simulink model "Model"  (R2024b)
settings: Solver=FixedStepAuto  StartTime=0.0  StopTime=17  FixedStep=0.001  RelTol=1e-3
values from neighbouring files (symbols this model uses):
  A_8 = 0.07    [Dane.m]
  C_Beta_vec = linspace(0, 1, beta_points)    [generate_maps.m]    (also in mapy_new.m = [0, 0.25, 0.5, 0.75, 1.0])
  C_Eff_map = zeros(n_points, beta_points)    [generate_maps.m]    (also in mapy_new.m = [)
  c_H = Ma*sqrt(R*kappa*T_H)    [Dane.m]
  C_Nc_vec = linspace(0.5, 1.05, n_points)    [generate_maps.m]    (also in mapy_new.m = [0.5, 0.8, 0.9, 1.0, 1.05])
  C_PR_map = zeros(n_points, beta_points)    [generate_maps.m]    (also in mapy_new.m = [)
  C_Wc_map = zeros(n_points, beta_points)    [generate_maps.m]    (also in mapy_new.m = [)
  cp = 1005    [Dane.m]
  cp_sp = 1152    [Dane.m]
  eta_c_nom = 0.78    [Dane.m]
  J = 5    [Dane.m]
  kappa = 1.4    [Dane.m]
  kappa_sp = 1.33    [Dane.m]
  m_dot_nom = 4.5    [Dane.m]
  Ma = 0.5    [Dane.m]
  n_nom = 41000    [Dane.m]
  p_0 = 101325    [Dane.m]
  p_H = p_0*(1-H/44300)^5.256    (= 53994.0459955)    [Dane.m]
  phi_d = 0.98    [Dane.m]
  pi_c_nom = 5.8    [Dane.m]
  pi_ks = 0.95    [Dane.m]
  R = 288    [Dane.m]
  sigma_rw = 1    [Dane.m]
  sigma_wl = 0.95    [Dane.m]
  T_0 = 288.15    [Dane.m]
  T_Eff_map = zeros(n_points, n_points)    [generate_maps.m]    (also in mapy_new.m = [)
  T_Nc_vec = linspace(0.5, 1.05, n_points)    [generate_maps.m]    (also in mapy_new.m = [0.5, 0.8, 0.9, 1.0, 1.05])
  T_PR_vec = linspace(1.2, 3.5, n_points)    [generate_maps.m]    (also in mapy_new.m = [1.5, 2.0, 2.5, 3.0, 3.5])
  T_Wc_map = zeros(n_points, n_points)    [generate_maps.m]    (also in mapy_new.m = [)
  W = 43*10^6    (= 43000000)    [Dane.m]
undefined symbols (not defined in the file or in its folder): m_dot
libraries: mpclib x1, slpidlib x1
settings Model: Creator=mordw  LastModifiedBy=mordw

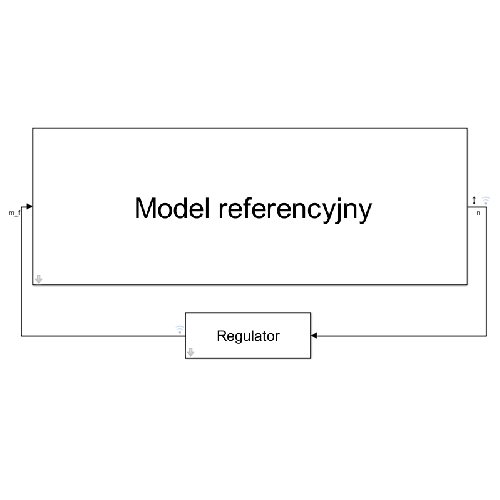
[thumbnail: Simulink's stored preview of the top-level diagram]
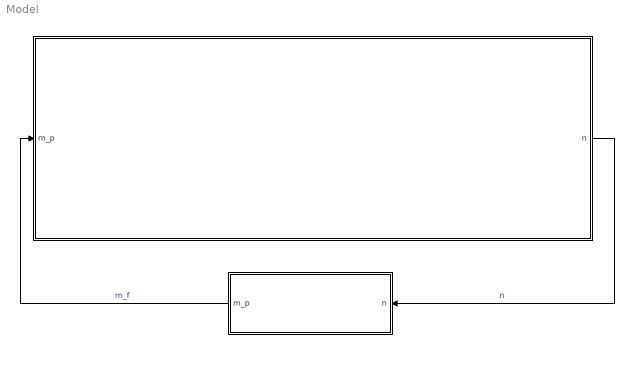
== system Model ==
  " " : Subsystem
      mask DialogControl Control2 Prompt: Reference model
  "  " : Subsystem
  wires:
  " "/1(n) -> "  "/1(n)  "n"
  "  "/1(m_p) -> " "/1(m_p)  "m_f"

== system Model/  ==
  m_p : Inport
  Reference dobry : Subsystem
  Terminator : Terminator  Commented=on
  Terminator1 : Terminator  Commented=on
  Terminator2 : Terminator  Commented=on
  n : Outport
  wires:
  m_p/1 -> Reference dobry/1(m_p1)
  Reference dobry/1(n1) -> n/1

== system Model/   ==
  n : Inport
  Constant : Constant  Commented=on  Value=n_nom
  Constant1 : Constant  Value=n_nom
  Constant2 : Constant
  MPC Controller : mpclib/MPC Controller  Commented=on  SCDEnableBlockLinearizationSpecification=on  mpcobj=mpc_controller  is_multiple=0  enable_value=0  return_u0=off  updateMPCinCallerWorkspace=on  md_inport=off  mv_inport=off  uref_inport=off  return_cost=off  return_mvseq=off  return_qpstatus=off  return_xseq=off  return_state=off  return_ovseq=off  state_inport=off  umin_inport=off  umax_inport=off  ymin_inport=off  ymax_inport=off  cc_inport=off  ywt_inport=off  uwt_inport=off  duwt_inport=off  rhoeps_inport=off  pm_inport=off  MaximumP=10  HorizonChoice=FixedHorizon  n_ts=0.01  n_p=50  n_mv=1  n_md=0  n_ud=0  n_mo=1  n_uo=0  BlockDataType=double  SampleTimeInherited=off  switch_inport=off
  PID Controller : slpidlib/PID Controller  Controller=PID  Form=Parallel  TimeDomain=Continuous-time  UseExternalTs=off  SampleTime=-1  IntegratorMethod=Forward Euler  FilterMethod=Forward Euler  ControllerParametersSource=internal  P=0.01  I=0.005  UseKiTs=off  D=0  UseExternalDerivativeSource=off  N=100  UseFilter=on  TunerSelectOption=Transfer Function Based (PID Tuner App)  InitialConditionSource=internal  InitialConditionForIntegrator=0  InitialConditionForFilter=0  DifferentiatorICPrevScaledInput=0  ExternalReset=none  TrackingMode=off  Kt=1  LimitOutput=on  SatLimitsSource=internal  UpperSaturationLimit=0.5  LowerSaturationLimit=0  LinearizeAsGain=on  AntiWindupMode=back-calculation  Kb=5  LimitIntegrator=off  UpperIntegratorSaturationLimit=inf  LowerIntegratorSaturationLimit=-inf  POutMin=[]  POutMax=[]  IOutMin=[]  IOutMax=[]  DOutMin=[]  DOutMax=[]  NOutMin=[]  NOutMax=[]  SumOutMin=[]  SumOutMax=[]  SaturationOutMin=[]  SaturationOutMax=[]  PParamMin=[]  PParamMax=[]  IParamMin=[]  IParamMax=[]  DParamMin=[]  DParamMax=[]  NParamMin=[]  NParamMax=[]  KbParamMin=[]  KbParamMax=[]  KtParamMin=[]  KtParamMax=[]  KbOutMin=[]  KbOutMax=[]  KtOutMin=[]  KtOutMax=[]  IntegratorOutMin=[]  IntegratorOutMax=[]  FilterOutMin=[]  FilterOutMax=[]  SumI1OutMin=[]  SumI1OutMax=[]  SumI2OutMin=[]  SumI2OutMax=[]  SumI3OutMin=[]  SumI3OutMax=[]  SumI4OutMin=[]  SumI4OutMax=[]  SumDOutMin=[]  SumDOutMax=[]  DifferentiatorOutMin=[]  DifferentiatorOutMax=[]  FilterDiffOutCoefMin=[]  FilterDiffOutCoefMax=[]  ReciprocalOutMin=[]  ReciprocalOutMax=[]  SumDenOutMin=[]  SumDenOutMax=[]  SumNumOutMin=[]  SumNumOutMax=[]  DivideOutMin=[]  DivideOutMax=[]  UdiffTsProdOutMin=[]  UdiffTsProdOutMax=[]  NTsProdOutMin=[]  NTsProdOutMax=[]  UintegralTsProdOutMin=[]  UintegralTsProdOutMax=[]  UngainTsProdOutMin=[]  UngainTsProdOutMax=[]  ClampingZeroOutDataTypeStr=Inherit: Inherit via back propagation  ClampingZeroOutMin=[]  ClampingZeroOutMax=[]  FilterDenConstantOutDataTypeStr=Inherit: Inherit via back propagation  FilterDenConstantOutMin=[]  FilterDenConstantOutMax=[]  PCopyOutDataTypeStr=Inherit: Inherit via back propagation  PCopyOutMin=[]  PCopyOutMax=[]  NCopyOutDataTypeStr=Inherit: Inherit via back propagation  NCopyOutMin=[]  NCopyOutMax=[]  IntegratorContinuousStateAttributes=''  IntegratorStateMustResolveToSignalObject=off  IntegratorRTWStateStorageClass=Auto  FilterContinuousStateAttributes=''  FilterStateMustResolveToSignalObject=off  FilterRTWStateStorageClass=Auto  ParallelPVariant=InternalParameters  IdealPVariant=Disabled  IVariant=InternalParameters  DVariant=InternalParameters  IntegratorVariant=Continuous  SatVariant=Enabled  AWVariant=BackCalculation  PCopyVariant=Disabled  TRVariant=Disabled  FdbkBlocksVariant=Forward  IdealPFdbkVariant=Disabled  SatFdbkVariant=Disabled  DerivativeFilterVariant=ContFilter  NVariant=InternalParameters  NCopyVariant=Disabled  FilterICVariant=InternalICsFilter  IntegratorICVariant=InternalICs  ExternalResetVariant=Disabled  TRSumVariant=Passthrough  SumFdbkVariant=Disabled  SumVariant=Sum_PID  TsampFilterVariant=InternalTs  TsampNgainVariant=Passthrough  TsampIntegralVariant=Disabled_SignalSpec  ExternalSaturationOutDataTypeStr=Inherit: Same as second input  DerivativeSourceVariant=ErrorSignal  PreIntVariant=InternalPreInt
  Sum : Sum  Inputs=|-+
  Switch : Switch  Criteria=u2 > Threshold  SaturateOnIntegerOverflow=off  InputSameDT=off
  m_p : Outport
  wires:
  n/1 -> Sum/1, MPC Controller/1
  PID Controller/1 -> Switch/1
  MPC Controller/1 -> Switch/3
  Constant1/1 -> Sum/2
  Constant/1 -> MPC Controller/2
  Sum/1 -> PID Controller/1
  Constant2/1 -> Switch/2
  Switch/1 -> m_p/1  "m_p"

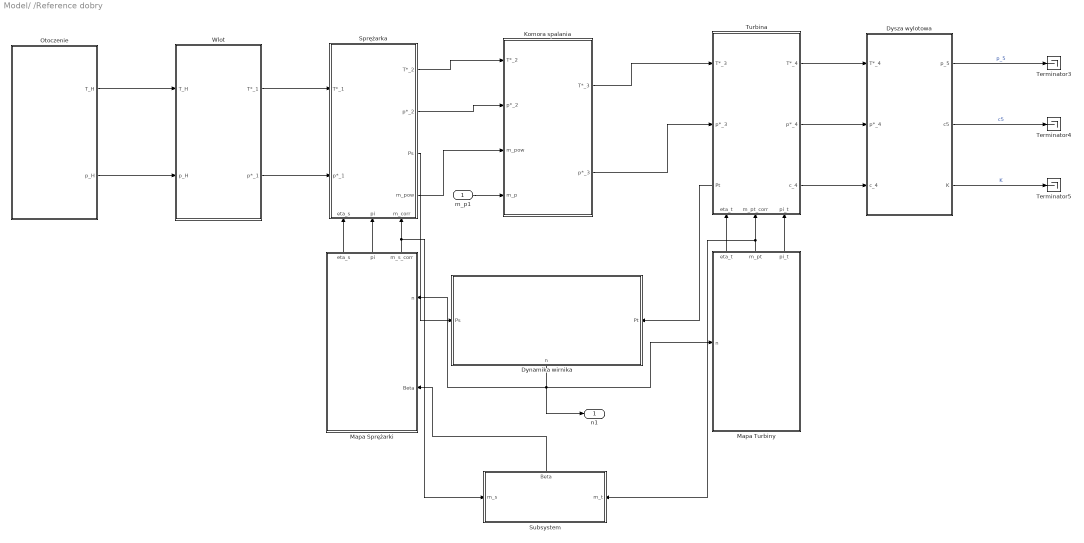
== system Model/ /Reference dobry ==
  m_p1 : Inport
  Dynamika wirnika : Subsystem
      settings: PortSchema="{\"entries\":[{\"content\":{\"sides\":[{\"content\":{\"connectorIds\":[\"In1\"]},\"type\":\"ConnectorPlacement.EquallySpacedRectSide\",\"uuid\":\"92648d91-603a-470e-8d2a-f02149c3db38\"},{\"content\":{\"connectorIds\":[\"In2\"],\"side\":\"RIGHT\"},\"type\":\"ConnectorPlacement.EquallySpacedRectSide\",\"uuid\":\"414f3566-06b2-4981-8d9f-99d3b0ae2fa9\"},{\"content\":{\"side\":\"TOP\"},\"type\":\"ConnectorPlacement.EquallySpacedRectSide\",\"uuid\":\"127541e1-5e00-46d2-b9c4-1484edc24234\"},{\"content\":{\"connectorIds\":[\"Out1\"],\"side\":\"BOTTOM\"},\"type\":\"ConnectorPlacement.EquallySpacedRectSide\",\"uuid\":\"a5106de6-ce0f-46b5-8051-6428c4816053\"}]},\"type\":\"ConnectorPlacement.EquallySpacedConnector\",\"uuid\":\"41cf9bbd-cf38-41c3-a622-f9a01faf9b59\"}],\"packageUris\":[\"http://schema.mathworks.com/mf0/Connector/R2020b\"],\"version\":\"1.0\"}"
  Dysza wylotowa : Subsystem
  Komora spalania : Subsystem
  Mapa Sprężarki : Subsystem
      settings: PortSchema="{\"entries\":[{\"content\":{\"sides\":[{\"content\":{},\"type\":\"ConnectorPlacement.EquallySpacedRectSide\",\"uuid\":\"8677f900-7922-4478-aeeb-e88a17ef6356\"},{\"content\":{\"connectorIds\":[\"In1\",\"In2\"],\"side\":\"RIGHT\"},\"type\":\"ConnectorPlacement.EquallySpacedRectSide\",\"uuid\":\"8ac603c2-697e-40fb-a61e-8eac1944f047\"},{\"content\":{\"connectorIds\":[\"Out1\",\"Out2\",\"Out3\"],\"side\":\"TOP\"},\"type\":\"ConnectorPlacement.EquallySpacedRectSide\",\"uuid\":\"1291509f-f986-4666-8166-1e03e99acc3f\"},{\"content\":{\"side\":\"BOTTOM\"},\"type\":\"ConnectorPlacement.EquallySpacedRectSide\",\"uuid\":\"87618aba-7d63-48a9-a830-8ed0b0805b31\"}]},\"type\":\"ConnectorPlacement.EquallySpacedConnector\",\"uuid\":\"5f7b5324-b2c0-4c4f-ba23-276b96a3be49\"}],\"packageUris\":[\"http://schema.mathworks.com/mf0/Connector/R2020b\"],\"version\":\"1.0\"}"
  Mapa Turbiny : Subsystem
      settings: PortSchema="{\"entries\":[{\"content\":{\"sides\":[{\"content\":{\"connectorIds\":[\"In1\"]},\"type\":\"ConnectorPlacement.EquallySpacedRectSide\",\"uuid\":\"5cf3ab21-3172-420e-8db2-451205a4f6d8\"},{\"content\":{\"side\":\"RIGHT\"},\"type\":\"ConnectorPlacement.EquallySpacedRectSide\",\"uuid\":\"e1f4544a-94e2-479d-8805-7e94a98bc078\"},{\"content\":{\"connectorIds\":[\"Out1\",\"Out2\",\"Out3\"],\"side\":\"TOP\"},\"type\":\"ConnectorPlacement.EquallySpacedRectSide\",\"uuid\":\"0d6b6710-b665-43c6-ac6f-8bcced33118f\"}]},\"type\":\"ConnectorPlacement.EquallySpacedConnector\",\"uuid\":\"393c9c26-fe71-43c8-a3ab-bf8cb9c23c8b\"}],\"packageUris\":[\"http://schema.mathworks.com/mf0/Connector/R2020b\"],\"version\":\"1.0\"}"
  Otoczenie : Subsystem
  Sprężarka : Subsystem
      settings: PortSchema="{\"entries\":[{\"content\":{\"sides\":[{\"content\":{\"connectorIds\":[\"In1\",\"In2\"]},\"type\":\"ConnectorPlacement.EquallySpacedRectSide\",\"uuid\":\"5ad9138f-573e-4bb6-8f90-45256150ad02\"},{\"content\":{\"connectorIds\":[\"Out1\",\"Out2\",\"Out3\",\"Out4\"],\"side\":\"RIGHT\"},\"type\":\"ConnectorPlacement.EquallySpacedRectSide\",\"uuid\":\"748e4777-2a7e-4826-9de5-35a340d0e0d9\"},{\"content\":{\"side\":\"TOP\"},\"type\":\"ConnectorPlacement.EquallySpacedRectSide\",\"uuid\":\"d6ba970d-5e85-4191-9407-cf63c790295c\"},{\"content\":{\"connectorIds\":[\"In3\",\"In4\",\"In5\"],\"side\":\"BOTTOM\"},\"type\":\"ConnectorPlacement.EquallySpacedRectSide\",\"uuid\":\"1930f8a7-28af-49c4-96e2-50b54aac2f51\"}]},\"type\":\"ConnectorPlacement.EquallySpacedConnector\",\"uuid\":\"98d1a612-9d3a-4741-82d1-8163c8f597bd\"}],\"packageUris\":[\"http://schema.mathworks.com/mf0/Connector/R2020b\"],\"version\":\"1.0\"}"
  Subsystem : Subsystem
      settings: PortSchema="{\"entries\":[{\"content\":{\"sides\":[{\"content\":{\"connectorIds\":[\"In1\"]},\"type\":\"ConnectorPlacement.EquallySpacedRectSide\",\"uuid\":\"a539ccee-3b56-4fd0-8aa8-8b3e66e9dd4a\"},{\"content\":{\"connectorIds\":[\"In2\"],\"side\":\"RIGHT\"},\"type\":\"ConnectorPlacement.EquallySpacedRectSide\",\"uuid\":\"8c1e68bc-092f-4324-808d-b2eeaf4424db\"},{\"content\":{\"connectorIds\":[\"Out1\"],\"side\":\"TOP\"},\"type\":\"ConnectorPlacement.EquallySpacedRectSide\",\"uuid\":\"5ad00f7f-de76-476d-96e9-8c0e667f1b36\"}]},\"type\":\"ConnectorPlacement.EquallySpacedConnector\",\"uuid\":\"625eb8fa-74b9-4e26-bcda-3b6095be352e\"}],\"packageUris\":[\"http://schema.mathworks.com/mf0/Connector/R2020b\"],\"version\":\"1.0\"}"
  Terminator3 : Terminator
  Terminator4 : Terminator
  Terminator5 : Terminator
  Turbina : Subsystem
      settings: PortSchema="{\"entries\":[{\"content\":{\"sides\":[{\"content\":{\"connectorIds\":[\"In1\",\"In2\",\"Out4\"]},\"type\":\"ConnectorPlacement.EquallySpacedRectSide\",\"uuid\":\"f4a9e5e5-b95d-47b8-93e5-cedd35d908d0\"},{\"content\":{\"connectorIds\":[\"Out1\",\"Out2\",\"Out3\"],\"side\":\"RIGHT\"},\"type\":\"ConnectorPlacement.EquallySpacedRectSide\",\"uuid\":\"10b6ea61-f01f-4e48-ad07-dc4cbfd91ff5\"},{\"content\":{\"side\":\"TOP\"},\"type\":\"ConnectorPlacement.EquallySpacedRectSide\",\"uuid\":\"208658a8-c4a1-42db-ac9c-b16758812c43\"},{\"content\":{\"connectorIds\":[\"In3\",\"In4\",\"In5\"],\"side\":\"BOTTOM\"},\"type\":\"ConnectorPlacement.EquallySpacedRectSide\",\"uuid\":\"fa42c5c3-0699-4620-9578-eed2ede52a20\"}]},\"type\":\"ConnectorPlacement.EquallySpacedConnector\",\"uuid\":\"0f96be96-72d8-41e4-aada-f9d1a25f1c70\"}],\"packageUris\":[\"http://schema.mathworks.com/mf0/Connector/R2020b\"],\"version\":\"1.0\"}"
  Wlot : Subsystem
  n1 : Outport
  wires:
  Komora spalania/2(p*_3) -> Turbina/2(p*_3)
  Komora spalania/1(T*_3) -> Turbina/1(T*_3)
  Mapa Turbiny/2(m_pt) -> Subsystem/2(m_t), Turbina/4(m_pt_corr)
  Otoczenie/2(p_H) -> Wlot/2(p_H)
  Dynamika wirnika/1(n) -> n1/1, Mapa Sprężarki/1(n), Mapa Turbiny/1(n)
  Turbina/4(Pt) -> Dynamika wirnika/2(Pt)
  Dysza wylotowa/2(c5) -> Terminator4/1  "c5"
  Mapa Turbiny/3(pi_t) -> Turbina/5(pi_t)
  Sprężarka/1(T*_2) -> Komora spalania/1(T*_2)
  Dysza wylotowa/1(p_5) -> Terminator3/1  "p_5"
  Mapa Sprężarki/2(pi) -> Sprężarka/4(pi)
  Dysza wylotowa/3(K) -> Terminator5/1  "K"
  Mapa Sprężarki/1(eta_s) -> Sprężarka/3(eta_s)
  Sprężarka/3(Ps) -> Dynamika wirnika/1(Ps)
  Turbina/3(c_4) -> Dysza wylotowa/3(c_4)
  Wlot/1(T*_1) -> Sprężarka/1(T*_1)
  Mapa Turbiny/1(eta_t) -> Turbina/3(eta_t)
  Turbina/1(T*_4) -> Dysza wylotowa/1(T*_4)
  Otoczenie/1(T_H) -> Wlot/1(T_H)
  Turbina/2(p*_4) -> Dysza wylotowa/2(p*_4)
  m_p1/1 -> Komora spalania/4(m_p)
  Wlot/2(p*_1) -> Sprężarka/2(p*_1)
  Sprężarka/2(p*_2) -> Komora spalania/2(p*_2)
  Mapa Sprężarki/3(m_s_corr) -> Subsystem/1(m_s), Sprężarka/5(m_corr)
  Sprężarka/4(m_pow) -> Komora spalania/3(m_pow)
  Subsystem/1(Beta) -> Mapa Sprężarki/2(Beta)

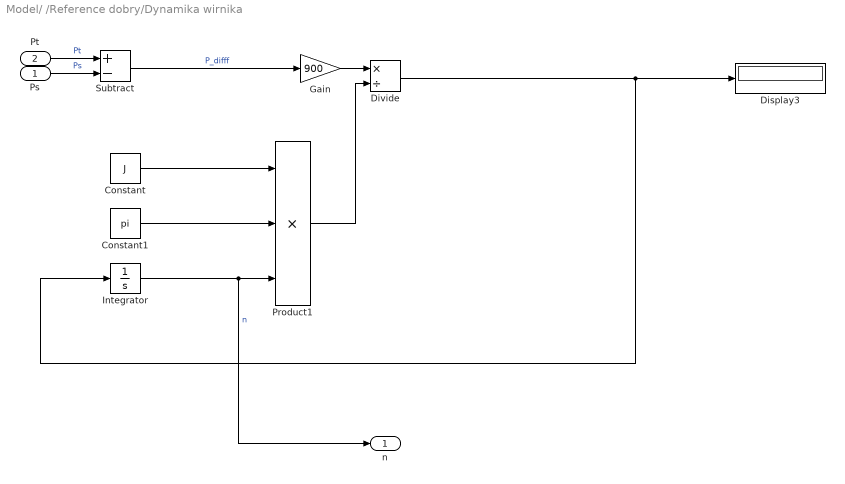
== system Model/ /Reference dobry/Dynamika wirnika ==
  Ps : Inport
  Pt : Inport  Port=2
  Constant : Constant  Value=J
  Constant1 : Constant  Value=pi
  Display3 : Display
  Divide : Product  Inputs=*/
  Gain : Gain  Gain=900
  Integrator : Integrator  InitialCondition=n_nom
  Product1 : Product  Inputs=3
  Subtract : Sum  Inputs=+-
  n : Outport
  wires:
  Integrator/1 -> n/1, Product1/3  "n"
  Divide/1 -> Integrator/1, Display3/1
  Pt/1 -> Subtract/1  "Pt"
  Subtract/1 -> Gain/1  "P_difff"
  Product1/1 -> Divide/2
  Constant1/1 -> Product1/2
  Constant/1 -> Product1/1
  Gain/1 -> Divide/1
  Ps/1 -> Subtract/2  "Ps"

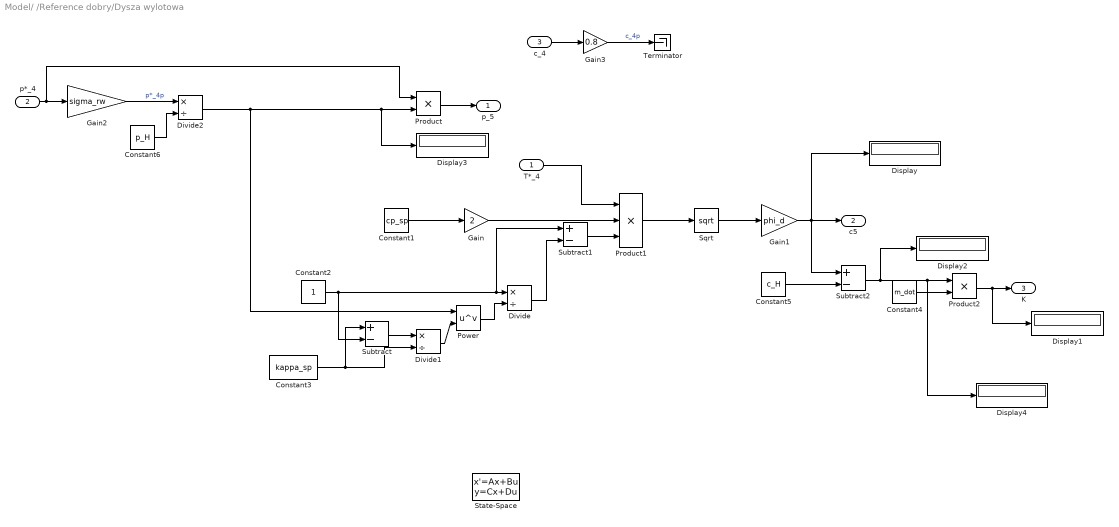
== system Model/ /Reference dobry/Dysza wylotowa ==
  T*_4 : Inport
  p*_4 : Inport  Port=2
  c_4 : Inport  Port=3
  Constant1 : Constant  Value=cp_sp
  Constant2 : Constant
  Constant3 : Constant  Value=kappa_sp
  Constant4 : Constant  Value=m_dot
  Constant5 : Constant  Value=c_H
  Constant6 : Constant  Value=p_H
  Display{,1..4} (5 alike) : Display
  Divide : Product  Inputs=*/
  Divide1 : Product  Inputs=*/
  Divide2 : Product  Inputs=*/
  Gain : Gain  Gain=2
  Gain1 : Gain  Gain=phi_d
  Gain2 : Gain  Gain=sigma_rw
  Gain3 : Gain  Gain=0.8
  Power : Math  Operator=pow
  Product : Product
  Product1 : Product  Inputs=3
  Product2 : Product
  Sqrt : Sqrt
  State-Space : StateSpace  InitialCondition=0
  Subtract : Sum  Inputs=+-
  Subtract1 : Sum  Inputs=+-
  Subtract2 : Sum  Inputs=+-
  Terminator : Terminator
  p_5 : Outport
  c5 : Outport  Port=2
  K : Outport  Port=3
  wires:
  Constant6/1 -> Divide2/2
  Gain3/1 -> Terminator/1  "c_4p"
  c_4/1 -> Gain3/1
  Gain2/1 -> Divide2/1  "p*_4p"
  Product2/1 -> K/1, Display1/1
  Subtract2/1 -> Product2/1, Display4/1, Display2/1
  Constant5/1 -> Subtract2/2
  Constant4/1 -> Product2/2
  Gain1/1 -> c5/1, Subtract2/1, Display/1
  Sqrt/1 -> Gain1/1
  Subtract1/1 -> Product1/3
  Divide/1 -> Subtract1/2
  Power/1 -> Divide/2
  Divide1/1 -> Power/2
  Subtract/1 -> Divide1/1
  Constant3/1 -> Subtract/1, Divide1/2
  Constant2/1 -> Subtract/2, Divide/1, Subtract1/1
  Product1/1 -> Sqrt/1
  T*_4/1 -> Product1/1
  Gain/1 -> Product1/2
  Constant1/1 -> Gain/1
  p*_4/1 -> Gain2/1, Product/1
  Divide2/1 -> Power/1, Product/2, Display3/1
  Product/1 -> p_5/1

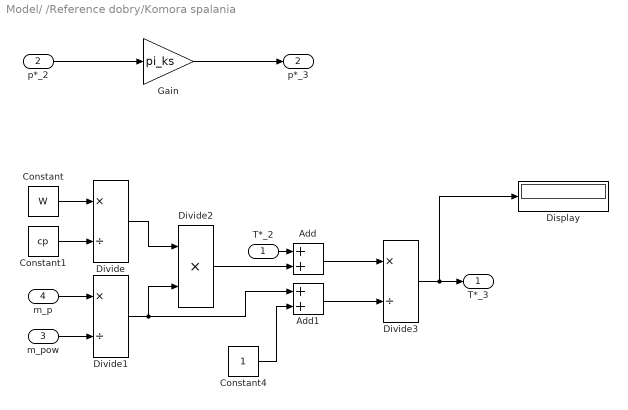
== system Model/ /Reference dobry/Komora spalania ==
  T*_2 : Inport
  p*_2 : Inport  Port=2
  m_pow : Inport  Port=3
  m_p : Inport  Port=4
  Add : Sum
  Add1 : Sum
  Constant : Constant  Value=W
  Constant1 : Constant  Value=cp
  Constant4 : Constant
  Display : Display
  Divide : Product  Inputs=*/
  Divide1 : Product  Inputs=*/
  Divide2 : Product  Inputs=**
  Divide3 : Product  Inputs=*/
  Gain : Gain  Gain=pi_ks
  T*_3 : Outport
  p*_3 : Outport  Port=2
  wires:
  m_p/1 -> Divide1/1
  Gain/1 -> p*_3/1
  p*_2/1 -> Gain/1
  Divide3/1 -> T*_3/1, Display/1
  Divide/1 -> Divide2/1
  Divide1/1 -> Divide2/2, Add1/1
  Constant4/1 -> Add1/2
  Add1/1 -> Divide3/2
  Add/1 -> Divide3/1
  T*_2/1 -> Add/1
  Divide2/1 -> Add/2
  m_pow/1 -> Divide1/2
  Constant1/1 -> Divide/2
  Constant/1 -> Divide/1

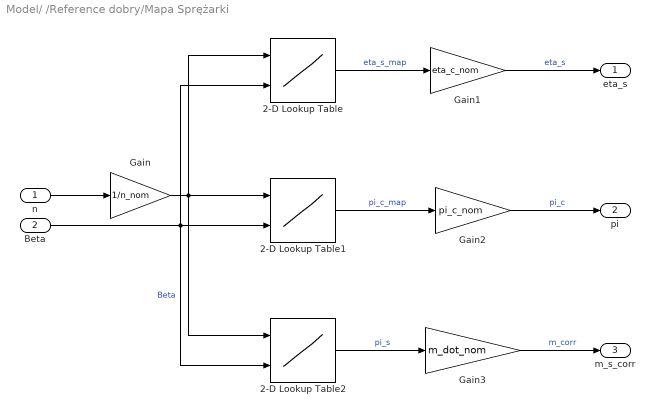
== system Model/ /Reference dobry/Mapa Sprężarki ==
  n : Inport
  Beta : Inport  Port=2
  2-D Lookup Table : Lookup_n-D  BreakpointsForDimension1=C_Nc_vec  BreakpointsForDimension2=C_Beta_vec  Table=C_Eff_map  InternalRulePriority=Speed  RndMeth=Simplest
      settings: InputPortMap=u0,u1
  2-D Lookup Table1 : Lookup_n-D  BreakpointsForDimension1=C_Nc_vec  BreakpointsForDimension2=C_Beta_vec  Table=C_PR_map  InternalRulePriority=Speed  RndMeth=Simplest
      settings: InputPortMap=u0,u1
  2-D Lookup Table2 : Lookup_n-D  BreakpointsForDimension1=C_Nc_vec  BreakpointsForDimension2=C_Beta_vec  Table=C_Wc_map  InternalRulePriority=Speed  RndMeth=Simplest
      settings: InputPortMap=u0,u1
  Gain : Gain  Gain=1/n_nom
  Gain1 : Gain  Gain=eta_c_nom
  Gain2 : Gain  Gain=pi_c_nom
  Gain3 : Gain  Gain=m_dot_nom
  eta_s : Outport
  pi : Outport  Port=2
  m_s_corr : Outport  Port=3
  wires:
  Gain/1 -> 2-D Lookup Table2/1, 2-D Lookup Table/1, 2-D Lookup Table1/1
  Beta/1 -> 2-D Lookup Table2/2, 2-D Lookup Table1/2, 2-D Lookup Table/2  "Beta"
  n/1 -> Gain/1
  2-D Lookup Table/1 -> Gain1/1  "eta_s_map"
  2-D Lookup Table1/1 -> Gain2/1  "pi_c_map"
  Gain1/1 -> eta_s/1  "eta_s"
  Gain2/1 -> pi/1  "pi_c"
  2-D Lookup Table2/1 -> Gain3/1  "pi_s"
  Gain3/1 -> m_s_corr/1  "m_corr"

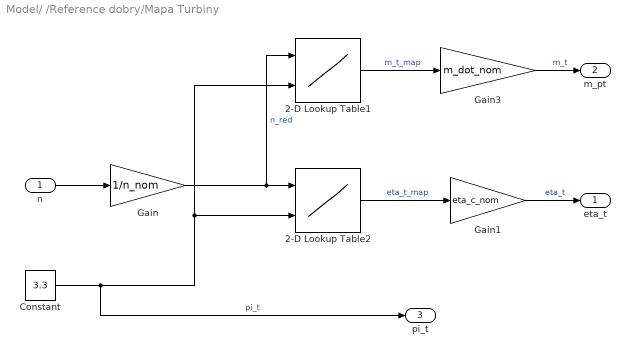
== system Model/ /Reference dobry/Mapa Turbiny ==
  n : Inport
  2-D Lookup Table1 : Lookup_n-D  BreakpointsForDimension1=T_Nc_vec  BreakpointsForDimension2=T_PR_vec  Table=T_Wc_map  InternalRulePriority=Speed  RndMeth=Simplest
      settings: InputPortMap=u0,u1
  2-D Lookup Table2 : Lookup_n-D  BreakpointsForDimension1=T_Nc_vec  BreakpointsForDimension2=T_PR_vec  Table=T_Eff_map  InternalRulePriority=Speed  RndMeth=Simplest
      settings: InputPortMap=u0,u1
  Constant : Constant  Value=3.3
  Gain : Gain  Gain=1/n_nom
  Gain1 : Gain  Gain=eta_c_nom
  Gain3 : Gain  Gain=m_dot_nom
  eta_t : Outport
  m_pt : Outport  Port=2
  pi_t : Outport  Port=3
  wires:
  2-D Lookup Table1/1 -> Gain3/1  "m_t_map"
  Gain/1 -> 2-D Lookup Table2/1, 2-D Lookup Table1/1  "n_red"
  2-D Lookup Table2/1 -> Gain1/1  "eta_t_map"
  n/1 -> Gain/1
  Constant/1 -> 2-D Lookup Table2/2, 2-D Lookup Table1/2, pi_t/1  "pi_t"
  Gain3/1 -> m_pt/1  "m_t"
  Gain1/1 -> eta_t/1  "eta_t"

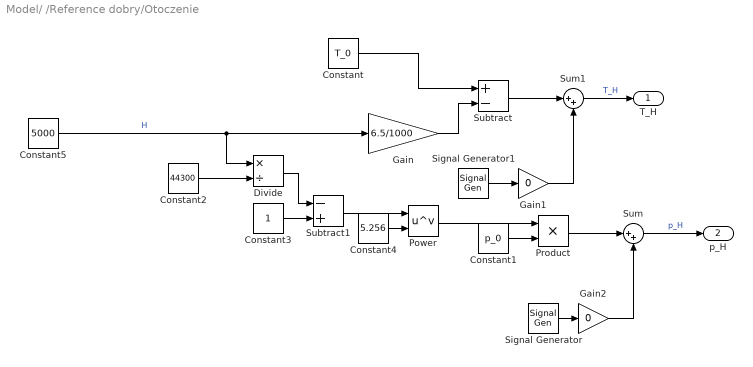
== system Model/ /Reference dobry/Otoczenie ==
  Constant : Constant  Value=T_0
  Constant1 : Constant  Value=p_0
  Constant2 : Constant  Value=44300
  Constant3 : Constant
  Constant4 : Constant  Value=5.256
  Constant5 : Constant  Value=5000
  Divide : Product  Inputs=*/
  Gain : Gain  Gain=6.5/1000
  Gain1 : Gain  Gain=0
  Gain2 : Gain  Gain=0
  Power : Math  Operator=pow
  Product : Product
  Signal Generator : SignalGenerator  WaveForm=square  Amplitude=5000  Frequency=0.5
  Signal Generator1 : SignalGenerator  Amplitude=15  Frequency=0.1
  Subtract : Sum  Inputs=+-
  Subtract1 : Sum  Inputs=-+
  Sum : Sum  Inputs=|++
  Sum1 : Sum  Inputs=|++
  T_H : Outport
  p_H : Outport  Port=2
  wires:
  Gain2/1 -> Sum/2
  Gain1/1 -> Sum1/2
  Sum1/1 -> T_H/1  "T_H"
  Signal Generator1/1 -> Gain1/1
  Signal Generator/1 -> Gain2/1
  Sum/1 -> p_H/1  "p_H"
  Constant4/1 -> Power/2
  Power/1 -> Product/1
  Product/1 -> Sum/1
  Subtract1/1 -> Power/1
  Constant3/1 -> Subtract1/2
  Constant2/1 -> Divide/2
  Divide/1 -> Subtract1/1
  Subtract/1 -> Sum1/1
  Constant/1 -> Subtract/1
  Gain/1 -> Subtract/2
  Constant5/1 -> Gain/1, Divide/1  "H"
  Constant1/1 -> Product/2

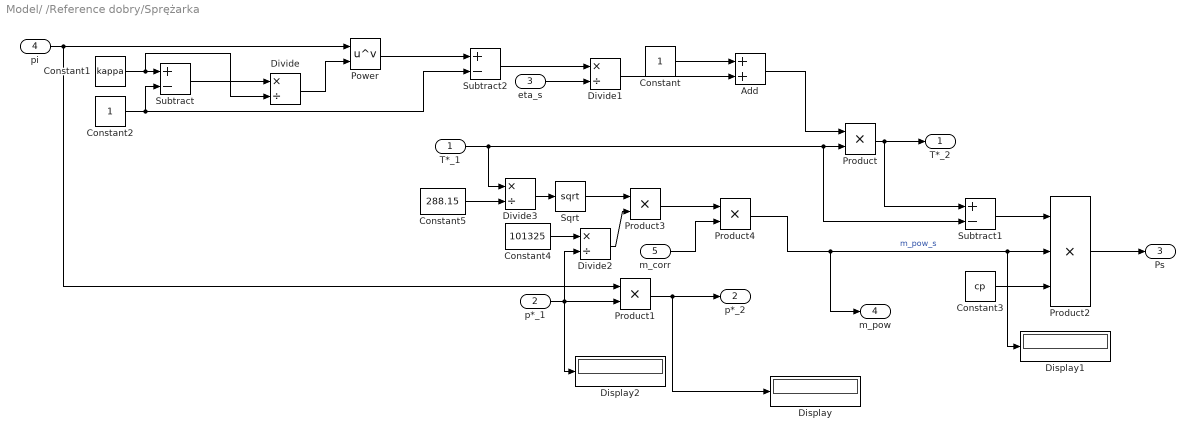
== system Model/ /Reference dobry/Sprężarka ==
  T*_1 : Inport
  p*_1 : Inport  Port=2
  eta_s : Inport  Port=3
  pi : Inport  Port=4
  m_corr : Inport  Port=5
  Add : Sum
  Constant : Constant
  Constant1 : Constant  Value=kappa
  Constant2 : Constant
  Constant3 : Constant  Value=cp
  Constant4 : Constant  Value=101325
  Constant5 : Constant  Value=288.15
  Display : Display
  Display1 : Display
  Display2 : Display
  Divide{,1..3} (4 alike) : Product  Inputs=*/
  Power : Math  Operator=pow
  Product{,1,3..4} (4 alike) : Product
  Product2 : Product  Inputs=3
  Sqrt : Sqrt
  Subtract : Sum  Inputs=+-
  Subtract1 : Sum  Inputs=+-
  Subtract2 : Sum  Inputs=+-
  T*_2 : Outport
  p*_2 : Outport  Port=2
  Ps : Outport  Port=3
  m_pow : Outport  Port=4
  wires:
  Constant3/1 -> Product2/3
  Product4/1 -> m_pow/1, Product2/2, Display1/1  "m_pow_s"
  Product2/1 -> Ps/1
  Subtract1/1 -> Product2/1
  Add/1 -> Product/1
  Constant/1 -> Add/1
  Divide1/1 -> Add/2
  eta_s/1 -> Divide1/2
  Subtract2/1 -> Divide1/1
  Product/1 -> T*_2/1, Subtract1/1
  Product1/1 -> p*_2/1, Display/1
  p*_1/1 -> Divide2/2, Display2/1, Product1/2
  T*_1/1 -> Subtract1/2, Product/2, Divide3/1
  Power/1 -> Subtract2/1
  Divide/1 -> Power/2
  Subtract/1 -> Divide/1
  Constant2/1 -> Subtract/2, Subtract2/2
  Constant1/1 -> Subtract/1, Divide/2
  pi/1 -> Power/1, Product1/1
  Constant4/1 -> Divide2/1
  Divide2/1 -> Product3/2
  Product3/1 -> Product4/1
  m_corr/1 -> Product4/2
  Constant5/1 -> Divide3/2
  Divide3/1 -> Sqrt/1
  Sqrt/1 -> Product3/1

== system Model/ /Reference dobry/Subsystem ==
  m_s : Inport
  m_t : Inport  Port=2
  Gain : Gain  Gain=m_dot_nom
  Gain1 : Gain  Gain=-1
  Integrator : Integrator  InitialCondition=1
  Saturation : Saturate  UpperLimit=1  LowerLimit=0.01
  Subtract : Sum  Inputs=+-
  Beta : Outport
  wires:
  m_s/1 -> Subtract/1  "m_c_corr"
  m_t/1 -> Subtract/2  "m_t_corr"
  Subtract/1 -> Gain/1
  Gain/1 -> Gain1/1
  Gain1/1 -> Integrator/1
  Integrator/1 -> Saturation/1
  Saturation/1 -> Beta/1  "Beta"

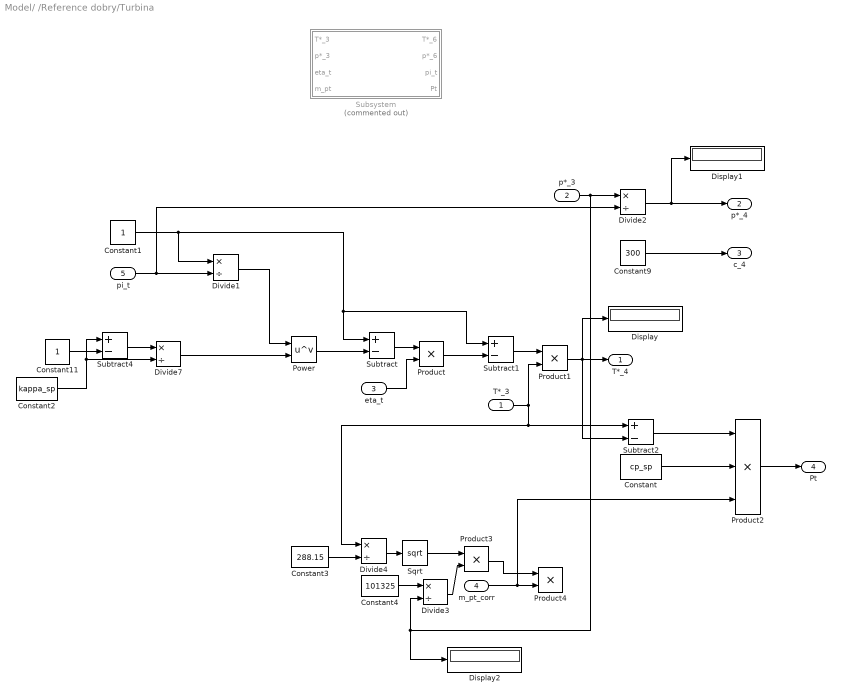
== system Model/ /Reference dobry/Turbina ==
  T*_3 : Inport
  p*_3 : Inport  Port=2
  eta_t : Inport  Port=3
  m_pt_corr : Inport  Port=4
  pi_t : Inport  Port=5
  Constant : Constant  Value=cp_sp
  Constant1 : Constant
  Constant11 : Constant
  Constant2 : Constant  Value=kappa_sp
  Constant3 : Constant  Value=288.15
  Constant4 : Constant  Value=101325
  Constant9 : Constant  Value=300
  Display : Display
  Display1 : Display
  Display2 : Display
  Divide{1..4,7} (5 alike) : Product  Inputs=*/
  Power : Math  Operator=pow
  Product{,1,3..4} (4 alike) : Product
  Product2 : Product  Inputs=3
  Sqrt : Sqrt
  Subsystem : Subsystem  Commented=on
  Subtract{,1..2,4} (4 alike) : Sum  Inputs=+-
  T*_4 : Outport
  p*_4 : Outport  Port=2
  c_4 : Outport  Port=3
  Pt : Outport  Port=4
  wires:
  Subtract2/1 -> Product2/1
  Constant/1 -> Product2/2
  Subtract1/1 -> Product1/1
  Product/1 -> Subtract1/2
  eta_t/1 -> Product/2
  Subtract/1 -> Product/1
  Power/1 -> Subtract/2
  Divide1/1 -> Power/1
  Constant1/1 -> Subtract/1, Subtract1/1, Divide1/1
  pi_t/1 -> Divide1/2, Divide2/2
  Constant2/1 -> Subtract4/1, Divide7/2
  Constant11/1 -> Subtract4/2
  Subtract4/1 -> Divide7/1
  Divide7/1 -> Power/2
  Product2/1 -> Pt/1
  Constant9/1 -> c_4/1
  Divide2/1 -> p*_4/1, Display1/1
  Product1/1 -> T*_4/1, Subtract2/2, Display/1
  Product3/1 -> Product4/1
  Divide4/1 -> Sqrt/1
  Sqrt/1 -> Product3/1
  Divide3/1 -> Product3/2
  m_pt_corr/1 -> Product2/3, Product4/2
  T*_3/1 -> Product1/2, Divide4/1, Subtract2/1
  p*_3/1 -> Divide3/2, Display2/1, Divide2/1
  Constant3/1 -> Divide4/2
  Constant4/1 -> Divide3/1

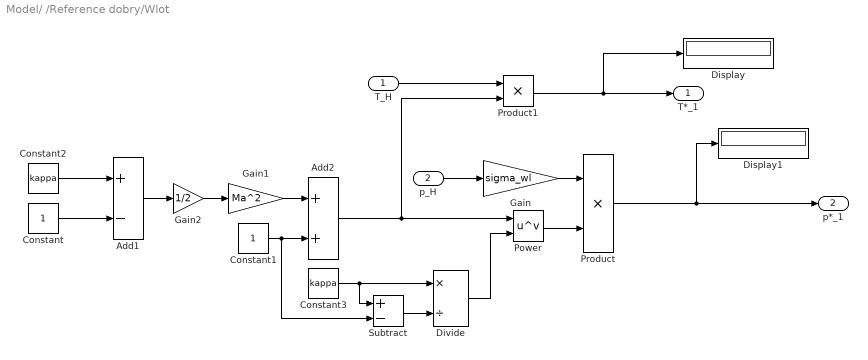
== system Model/ /Reference dobry/Wlot ==
  T_H : Inport
  p_H : Inport  Port=2
  Add1 : Sum  Inputs=+-
  Add2 : Sum
  Constant : Constant
  Constant1 : Constant
  Constant2 : Constant  Value=kappa
  Constant3 : Constant  Value=kappa
  Display : Display
  Display1 : Display
  Divide : Product  Inputs=*/
  Gain : Gain  Gain=sigma_wl
  Gain1 : Gain  Gain=Ma^2
  Gain2 : Gain  Gain=1/2
  Power : Math  Operator=pow
  Product : Product
  Product1 : Product
  Subtract : Sum  Inputs=+-
  T*_1 : Outport
  p*_1 : Outport  Port=2
  wires:
  Product1/1 -> Display/1, T*_1/1
  T_H/1 -> Product1/1
  Gain2/1 -> Gain1/1
  Product/1 -> Display1/1, p*_1/1
  Power/1 -> Product/2
  Divide/1 -> Power/2
  Subtract/1 -> Divide/2
  Constant3/1 -> Subtract/1, Divide/1
  Constant1/1 -> Add2/2, Subtract/2
  Gain1/1 -> Add2/1
  Add1/1 -> Gain2/1
  Constant2/1 -> Add1/1
  Constant/1 -> Add1/2
  Gain/1 -> Product/1
  p_H/1 -> Gain/1
  Add2/1 -> Power/1, Product1/2

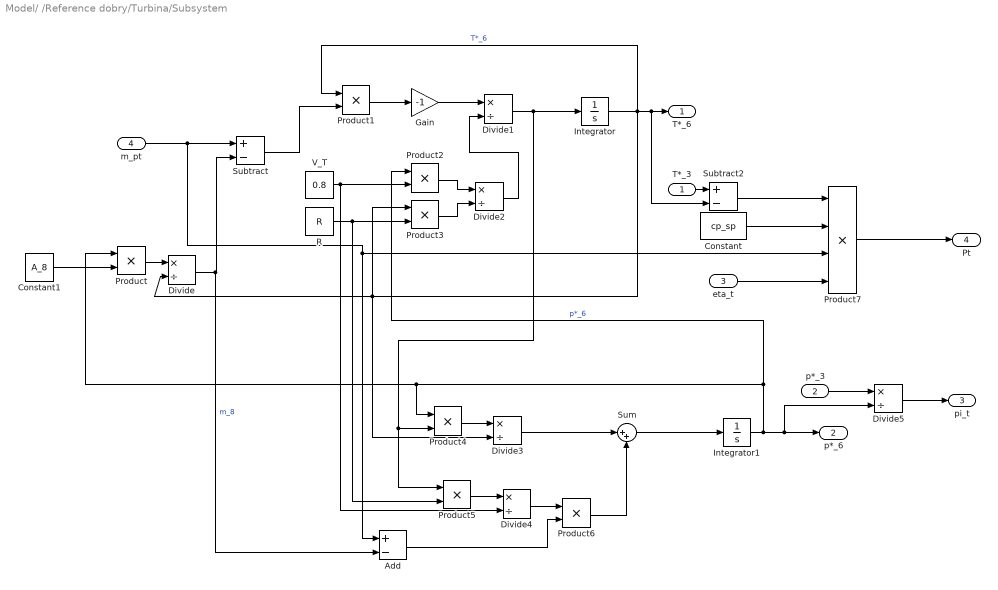
== system Model/ /Reference dobry/Turbina/Subsystem ==
  T*_3 : Inport
  p*_3 : Inport  Port=2
  eta_t : Inport  Port=3
  m_pt : Inport  Port=4
  Add : Sum  Inputs=+-
  Constant : Constant  Value=cp_sp
  Constant1 : Constant  Value=A_8
  Divide{,1..5} (6 alike) : Product  Inputs=*/
  Gain : Gain  Gain=-1
  Integrator : Integrator  InitialCondition=600
  Integrator1 : Integrator  InitialCondition=90000  UpperSaturationLimit=200000  LowerSaturationLimit=0
  Product{,1..6} (7 alike) : Product
  Product7 : Product  Inputs=4
  R : Constant  Value=R
  Subtract : Sum  Inputs=+-
  Subtract2 : Sum  Inputs=+-
  Sum : Sum  Inputs=|++
  V_T : Constant  Value=0.8
  T*_6 : Outport
  p*_6 : Outport  Port=2
  pi_t : Outport  Port=3
  Pt : Outport  Port=4
  wires:
  T*_3/1 -> Subtract2/1
  Sum/1 -> Integrator1/1
  eta_t/1 -> Product7/4
  Gain/1 -> Divide1/1
  Subtract2/1 -> Product7/1
  Constant/1 -> Product7/2
  Add/1 -> Product6/2
  Integrator/1 -> Divide3/2, Product3/1, Divide/2, Product1/1, Subtract2/2, T*_6/1  "T*_6"
  Subtract/1 -> Product1/2
  Product3/1 -> Divide2/2
  Divide/1 -> Add/2, Subtract/2  "m_8"
  Product4/1 -> Divide3/1
  p*_3/1 -> Divide5/1
  Product7/1 -> Pt/1
  Divide4/1 -> Product6/1
  Integrator1/1 -> Product2/1, Product/1, Product4/1, Divide5/2, p*_6/1  "p*_6"
  Divide3/1 -> Sum/1
  R/1 -> Product5/2, Product3/2
  Divide5/1 -> pi_t/1
  Divide1/1 -> Product5/1, Product4/2, Integrator/1
  Product1/1 -> Gain/1
  Product2/1 -> Divide2/1
  m_pt/1 -> Add/1, Product7/3, Subtract/1
  Divide2/1 -> Divide1/2
  V_T/1 -> Divide4/2, Product2/2
  Product5/1 -> Divide4/1
  Constant1/1 -> Product/2
  Product6/1 -> Sum/2
  Product/1 -> Divide/1
